simulink model "L11_Model"  (R2020b)
settings: Solver=VariableStepAuto  StartTime=0.0  StopTime=10000.0  RelTol=1e-3
values from neighbouring files (symbols this model uses):
  a = 0.9    [L11.m]
settings Model: Creator=Nic  LastModifiedBy=Nic

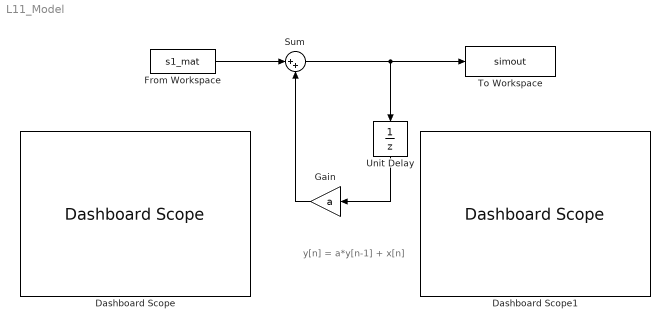
== system L11_Model ==
  note: y[n] = a*y[n-1] + x[n]
  Dashboard Scope : DashboardScope
  Dashboard Scope1 : DashboardScope
  From Workspace : FromWorkspace  VariableName=s1_mat  SampleTime=1
  Gain : Gain  Gain=a
  Sum : Sum  Inputs=|++
  To Workspace : ToWorkspace  VariableName=simout  SampleTime=-1
  Unit Delay : UnitDelay  SampleTime=-1  HasFrameUpgradeWarning=on
  wires:
  From Workspace/1 -> Sum/1
  Gain/1 -> Sum/2
  Unit Delay/1 -> Gain/1
  Sum/1 -> To Workspace/1, Unit Delay/1
